simulink model "QubeServo3Disk_Workspace"  (R2023a)
settings: Solver=ode4  StartTime=0.0  StopTime=inf  FixedStep=1/1000  RelTol=1e-3  EnableMultiTasking=on
libraries: quarc_library x6, simulink x5
settings Model: SimulationMode=external  ExtModeTrigDuration=10000  Creator=mbohra  LastModifiedBy=mbohra
settings SolverCC: AlgebraicLoopSolver=TrustRegion  PositivePriorityOrder=on
settings DataIOCC: ReturnWorkspaceOutputs=off
settings OptimizationCC: ReuseModelBlockBuffer=off
settings DebuggingCC: UnconnectedInputMsg=warning  UnconnectedOutputMsg=warning  UnconnectedLineMsg=warning  ArithmeticOperatorsInVariantConditions=warning
settings ModelReferenceCC: EnableRefExpFcnMdlSchedulingChecks=on
settings SFSimCC: SimUseLocalCustomCode=off  CustomCodeUndefinedFunction=UseInterfaceOnly
settings RTWCC: Description=QUARC Win64 Target Using Toolchain  SystemTargetFile=quarc_win64.tlc  TemplateMakefile=quarc_default_tmf  RTWUseLocalCustomCode=off  Toolchain=QUARC win64 | nmake (64-bit Windows)  BuildConfiguration=Faster Runs  DLArmComputeVersion=19.05
settings CodeAppCC: StateflowObjectComments=on
settings STFCustomTargetCC: SystemTargetFile=quarc_win64.tlc
settings GRTTargetCC: ParMdlRefBuildCompliant=off  CompOptLevelCompliant=off  CombineOutputUpdateFcns=off  MatFileLogging=off  CPPClassGenCompliant=off  GRTInterface=on  ExtMode=on  ExtModeMexFile=quarc_comm
settings ConfigComp: CovMetricSettings=dswe

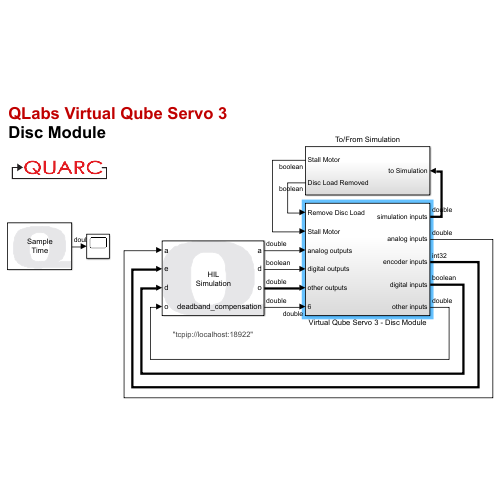
[thumbnail: Simulink's stored preview of the top-level diagram]
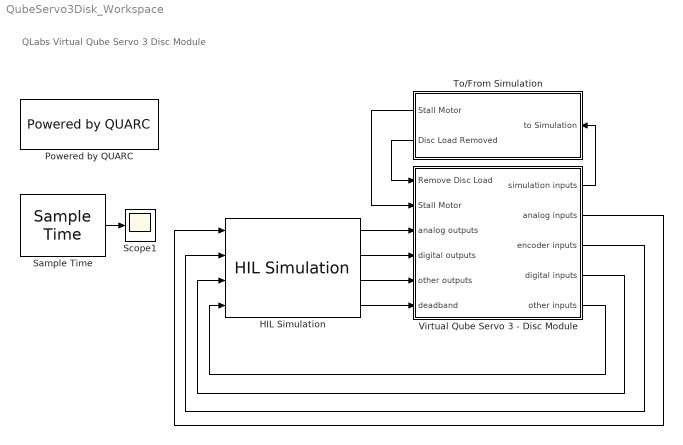
== system QubeServo3Disk_Workspace ==
  note: QLabs Virtual Qube Servo 3
      | Disc Module
  HIL Simulation : quarc_library/Data Acquisition/Generic/Configuration/HIL Simulation  uri_source=Specify via dialog (do not evaluate)  uri=tcpip://localhost:18922  board_type=qube_servo3_usb  board_id=0  options=deadband_compensation=%f[0,0.70]  sample_time=qc_get_step_size  active=on  num_clocks=1  num_interrupts=0  num_analog_inputs=1  num_analog_outputs=1  initial_analog=[]  num_digital_io=0  num_digital_inputs=3  num_digital_outputs=1  initial_digital=[]  num_encoder_inputs=2  num_pwm_outputs=0  initial_pwm=[]  other_inputs=[14000]  other_outputs=[11000:11002]  initial_other=[]  integer_get_property_codes=[]  double_get_property_codes=[]  string_get_property_codes=[]  integer_set_property_codes=[]  double_set_property_codes=[]  string_set_property_codes=[]  initial_integer_properties=0  initial_double_properties=0  max_string_property=80  use_variable_size_strings=off
      settings: AttributesFormatString="\"tcpip://localhost:18922\""  SourceProductName=QUARC Targets
  Powered by QUARC : quarc_library/Logos/Powered by QUARC
  Sample Time : quarc_library/Sources/Time/Sample Time  Priority=-99  sample_time=qc_get_step_size
  Scope1 : Scope
  To/From Simulation : Subsystem
  Virtual Qube Servo 3 - Disc Module : Subsystem
  wires:
  Sample Time/1 -> Scope1/1
  Virtual Qube Servo 3 - Disc Module/1(simulation inputs) -> To/From Simulation/1(to Simulation)
  HIL Simulation/1 -> Virtual Qube Servo 3 - Disc Module/3(analog outputs)
  HIL Simulation/2 -> Virtual Qube Servo 3 - Disc Module/4(digital outputs)
  Virtual Qube Servo 3 - Disc Module/2(analog inputs) -> HIL Simulation/1
  Virtual Qube Servo 3 - Disc Module/5(other inputs) -> HIL Simulation/4
  Virtual Qube Servo 3 - Disc Module/3(encoder inputs) -> HIL Simulation/2
  Virtual Qube Servo 3 - Disc Module/4(digital inputs) -> HIL Simulation/3
  To/From Simulation/2(Disc Load Removed) -> Virtual Qube Servo 3 - Disc Module/1(Remove Disc Load)
  To/From Simulation/1(Stall Motor) -> Virtual Qube Servo 3 - Disc Module/2(Stall Motor)
  HIL Simulation/3 -> Virtual Qube Servo 3 - Disc Module/5(other outputs)
  HIL Simulation/4 -> Virtual Qube Servo 3 - Disc Module/6(deadband)

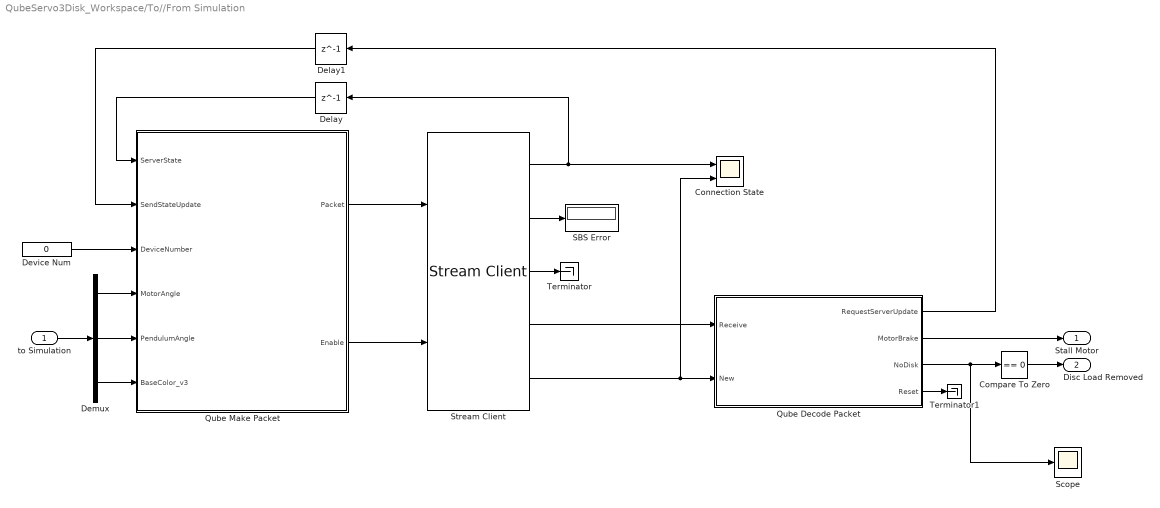
== system QubeServo3Disk_Workspace/To//From Simulation ==
  to Simulation : Inport
  Compare To Zero : simulink/Logic and Bit Operations/Compare To Zero  relop===  OutDataTypeStr=boolean
  "Connection State " : Scope  NumInputPorts=2
  Delay : Delay  DelayLength=1
  Delay1 : Delay  DelayLength=1
  Demux : Demux  Outputs=[1,1,3]
  Device Num : Constant  Value=0
  Qube Decode Packet : MATLAB Function  TreatAsAtomicUnit=on
  Qube Make Packet : MATLAB Function  TreatAsAtomicUnit=on
  SBS Error : Display
  Scope : Scope
  Stream Client : quarc_library/Communications/Basic/Stream Client  uri_source=Specify via dialog (do not evaluate)  uri=tcpip://localhost:18000?nagle='off'  send_buffer_size=65537  receive_buffer_size=65537  byte_order=little endian (Intel - LSB first)  optimization=Minimum latency  send_options=Send all data  receive_options=Receive all data  default_value=[0]  sample_time=qc_get_step_size  active=off  implementation=Use blocking I/O in a separate thread  send_fifo_size=3  receive_fifo_size=3  send_priority=0  receive_priority=0  send_dimensions=on  receive_dimensions=on  max_dimensions=65537  data_type=uint8  type_expr=BusObject
      settings: AttributesFormatString="\"tcpip://localhost:18000?nagle='off'\""
  Terminator : Terminator
  Terminator1 : Terminator
  Stall Motor : Outport  VectorParamsAs1DForOutWhenUnconnected=off
  Disc Load Removed : Outport  Port=2  VectorParamsAs1DForOutWhenUnconnected=off
  wires:
  Stream Client/4 -> Qube Decode Packet/1(Receive)
  Stream Client/5 -> "Connection State "/2, Qube Decode Packet/2(New)
  Stream Client/2 -> SBS Error/1
  Qube Decode Packet/1(RequestServerUpdate) -> Delay1/1
  Stream Client/3 -> Terminator/1
  Device Num/1 -> Qube Make Packet/3(DeviceNumber)
  Delay1/1 -> Qube Make Packet/2(SendStateUpdate)
  Delay/1 -> Qube Make Packet/1(ServerState)
  Stream Client/1 -> Delay/1, "Connection State "/1
  Qube Make Packet/1(Packet) -> Stream Client/1
  Qube Make Packet/2(Enable) -> Stream Client/2
  to Simulation/1 -> Demux/1
  Demux/1 -> Qube Make Packet/4(MotorAngle)
  Demux/2 -> Qube Make Packet/5(PendulumAngle)
  Demux/3 -> Qube Make Packet/6(BaseColor_v3)
  Qube Decode Packet/3(NoDisk) -> Scope/1, Compare To Zero/1
  Qube Decode Packet/4(Reset) -> Terminator1/1
  Qube Decode Packet/2(MotorBrake) -> Stall Motor/1
  Compare To Zero/1 -> Disc Load Removed/1

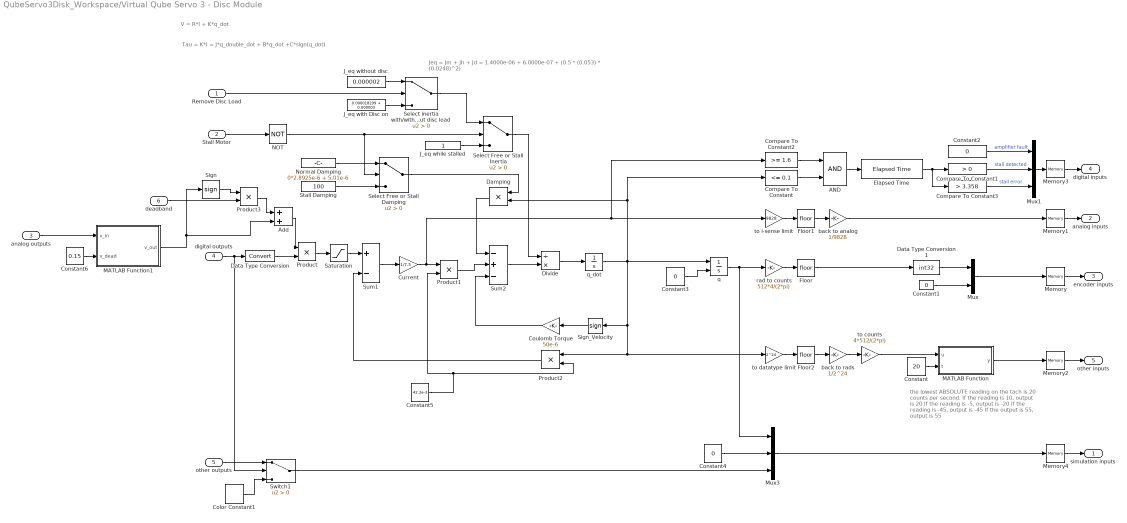
== system QubeServo3Disk_Workspace/Virtual Qube Servo 3 - Disc Module ==
  note: Jeq 		= Jm + Jh + Jd
      | 		= 1.4000e-06  +  6.0000e-07  +  (0.5 * (0.053) * (0.0248)^2)
  note: the lowest ABSOLUTE reading on the tach
      | is 20 counts per second.
      |
      | If the reading is 10, output is 20
      | If the reading is -5, output is -20
      | If the reading is -45, output is -45
      | If the output is 55, output is 55
  note: Tau = K*I = J*q_double_dot + B*q_dot +C*sign(q_dot)
  note: V = R*I + K*q_dot
  Remove Disc Load : Inport
  Stall Motor : Inport  Port=2
  analog outputs : Inport  Port=3
  digital outputs : Inport  Port=4
  other outputs : Inport  Port=5
  deadband : Inport  Port=6
  AND : Logic  AllPortsSameDT=off  OutDataTypeStr=boolean
  Add : Sum
  Color Constant1 : quarc_library/Sources/Signals/Color Constant  color=[1 0 0]
      settings: SourceProductName=QUARC Targets
  Compare To Constant : simulink/Logic and Bit Operations/Compare To Constant  relop=<=  const=0.1  OutDataTypeStr=boolean
  Compare To Constant1 : simulink/Logic and Bit Operations/Compare To Constant  relop=>  const=0  OutDataTypeStr=boolean
  Compare To Constant2 : simulink/Logic and Bit Operations/Compare To Constant  relop=>=  const=1.6  OutDataTypeStr=boolean
  Compare To Constant3 : simulink/Logic and Bit Operations/Compare To Constant  relop=>  const=3.358  OutDataTypeStr=boolean
  Constant : Constant  Value=20
  Constant1 : Constant  Value=0  OutDataTypeStr=int32
  Constant2 : Constant  Value=0  OutDataTypeStr=Inherit: Inherit via back propagation
  Constant3 : Constant  Value=0
  Constant4 : Constant  Value=0
  Constant5 : Constant  Value=42.2e-3
  Constant6 : Constant  Value=0.15
  Coulomb Torque : Gain  Gain=50e-6
  Current : Gain  Gain=1/7.5
  Damping : Product
  Data Type Conversion : DataTypeConversion  SaturateOnIntegerOverflow=off  RndMeth=Floor
  Data Type Conversion1 : DataTypeConversion  OutDataTypeStr=int32  SaturateOnIntegerOverflow=off  RndMeth=Floor
  Divide : Product  Inputs=/*
  Elapsed Time : quarc_library/Advanced/Timing/Elapsed Time  start_src=on  sample_time=-1
      settings: SourceProductName=QUARC Targets
  Floor : Rounding
  Floor1 : Rounding
  Floor2 : Rounding
  J_eq while stalled : Constant
  "J_eq with Disc on " : Constant  Value=0.000018299 + 0.000003
  J_eq without disc : Constant  Value=0.000002
  MATLAB Function : MATLAB Function  TreatAsAtomicUnit=on
  MATLAB Function1 : MATLAB Function  TreatAsAtomicUnit=on
  Memory : Memory  InitialCondition=[0 0]  InheritSampleTime=on
  Memory1 : Memory
  Memory2 : Memory
  Memory3 : Memory  InitialCondition=[0 0 0]
  Memory4 : Memory  InitialCondition=[0 0 1 0 0]
  Mux : Mux  Inputs=2
  Mux1 : Mux  Inputs=3
  Mux3 : Mux  Inputs=3
  NOT : Logic  Operator=NOT  IconShape=distinctive  AllPortsSameDT=off  OutDataTypeStr=boolean
  Normal Damping : Constant  Value=0*2.8925e-6 + 5.01e-6
  Product{,1..3} (4 alike) : Product
  Saturation : Saturate  UpperLimit=15  LowerLimit=-15
  Select Free or Stall Damping : Switch  Criteria=u2 > Threshold  SaturateOnIntegerOverflow=off  InputSameDT=off
  Select Free or Stall Inertia : Switch  Criteria=u2 > Threshold  SaturateOnIntegerOverflow=off  InputSameDT=off
  Select inertia with/without disc load : Switch  Criteria=u2 > Threshold  SaturateOnIntegerOverflow=off  InputSameDT=off
  Sign : Signum
  Sign_Velocity : Signum
  Stall Damping : Constant  Value=100
  Sum1 : Sum  Inputs=+-
  Sum2 : Sum  Inputs=-+-
  Switch1 : Switch  Criteria=u2 > Threshold  SaturateOnIntegerOverflow=off  InputSameDT=off
  back to rads : Gain  Gain=1/2^24
  back to analog : Gain  Gain=1/9828
  q : Integrator  ExternalReset=either
  q_dot : Integrator
  rad to counts : Gain  Gain=512*4/(2*pi)
  to counts : Gain  Gain=4*512/(2*pi)
  to datatype limit : Gain  Gain=2^24
  to i-sense limit : Gain  Gain=9828
  simulation inputs : Outport  VectorParamsAs1DForOutWhenUnconnected=off
  analog inputs : Outport  Port=2  VectorParamsAs1DForOutWhenUnconnected=off
  encoder inputs : Outport  Port=3  VectorParamsAs1DForOutWhenUnconnected=off
  digital inputs : Outport  Port=4  VectorParamsAs1DForOutWhenUnconnected=off
  other inputs : Outport  Port=5  VectorParamsAs1DForOutWhenUnconnected=off
  wires:
  digital outputs/1 -> Switch1/2, Data Type Conversion/1
  rad to counts/1 -> Floor/1
  q/1 -> Mux3/1, rad to counts/1
  Mux/1 -> Memory/1
  Constant1/1 -> Mux/2
  Data Type Conversion/1 -> Product/2
  Data Type Conversion1/1 -> Mux/1
  Memory/1 -> encoder inputs/1
  Memory1/1 -> analog inputs/1
  Memory2/1 -> other inputs/1
  Mux1/1 -> Memory3/1
  Compare To Constant/1 -> AND/2
  Compare To Constant2/1 -> AND/1
  AND/1 -> Elapsed Time/1
  Elapsed Time/1 -> Compare To Constant1/1, Compare To Constant3/1
  Compare To Constant1/1 -> Mux1/2  "stall detected"
  Compare To Constant3/1 -> Mux1/3  "stall error"
  Constant2/1 -> Mux1/1  "amplifier fault"
  Memory3/1 -> digital inputs/1
  Floor/1 -> Data Type Conversion1/1
  to counts/1 -> MATLAB Function/1(u)
  to datatype limit/1 -> Floor2/1
  Floor2/1 -> back to rads/1
  back to rads/1 -> to counts/1
  MATLAB Function/1(y) -> Memory2/1
  to i-sense limit/1 -> Floor1/1
  Floor1/1 -> back to analog/1
  back to analog/1 -> Memory1/1
  Constant/1 -> MATLAB Function/2(t)
  Constant3/1 -> q/2
  Saturation/1 -> Sum1/1
  q_dot/1 -> Compare To Constant/1, Damping/2, Product2/1, to datatype limit/1, Sign_Velocity/1, q/1
  Sum2/1 -> Divide/2
  Coulomb Torque/1 -> Sum2/3
  Divide/1 -> q_dot/1
  Sign_Velocity/1 -> Coulomb Torque/1
  Product2/1 -> Sum1/2
  Current/1 -> Product1/1, to i-sense limit/1, Compare To Constant2/1
  Product/1 -> Saturation/1
  Sum1/1 -> Current/1
  Product1/1 -> Sum2/2
  Select inertia with/without disc load/1 -> Select Free or Stall Inertia/1
  Stall Motor/1 -> NOT/1
  J_eq while stalled/1 -> Select Free or Stall Inertia/3
  J_eq without disc/1 -> Select inertia with/without disc load/1
  "J_eq with Disc on "/1 -> Select inertia with/without disc load/3
  Select Free or Stall Inertia/1 -> Divide/1
  other outputs/1 -> Switch1/1
  Constant4/1 -> Mux3/2
  Mux3/1 -> Memory4/1
  Color Constant1/1 -> Switch1/3
  Memory4/1 -> simulation inputs/1
  Switch1/1 -> Mux3/3
  Damping/1 -> Sum2/1
  Stall Damping/1 -> Select Free or Stall Damping/3
  Normal Damping/1 -> Select Free or Stall Damping/1
  Select Free or Stall Damping/1 -> Damping/1
  NOT/1 -> Select Free or Stall Damping/2, Select Free or Stall Inertia/2
  Constant5/1 -> Product2/2, Product1/2
  MATLAB Function1/1(v_out) -> Add/2, Sign/1
  Sign/1 -> Product3/1
  deadband/1 -> Product3/2
  Product3/1 -> Add/1
  Add/1 -> Product/1
  Remove Disc Load/1 -> Select inertia with/without disc load/2
  Constant6/1 -> MATLAB Function1/2(v_dead)
  analog outputs/1 -> MATLAB Function1/1(v_in)

== matlab function QubeServo3Disk_Workspace/To//From Simulation/Qube Make Packet ==
  settings: updateMethod=DISCRETE  sampleTime=qc_get_step_size
  data: Packet output size=65537; ServerState input; SendStateUpdate input; Enable output; DeviceNumber input; MotorAngle input; PendulumAngle input; BaseColor_v3 input
function [Packet,Enable] = QubeMakePacket(ServerState, SendStateUpdate, DeviceNumber, MotorAngle, PendulumAngle, BaseColor_v3) 

% Be sure to set the maximum signal size of the variable size Packet port 
% in Simulink->Edit Data of the editor window.  Size should be 65537 or
% larger to ensure that the stream server generates a 4 byte packet size.

%% Setup
persistent LastServerState;

if isempty(LastServerState)
    LastServerState = uint8(0);
end

Enable = 0;
Packet = uint8([]);

%% On connection
if ((ServerState == 2) && (LastServerState ~= 2))
    Packet = Qube3MakeCommandStateContainer(DeviceNumber, MotorAngle, PendulumAngle, BaseColor_v3); 
    Packet = [Packet; Qube3MakeModeRequestContainer(DeviceNumber)];
end

%% Send new State Container
% Previous state processed, send a new one
if (SendStateUpdate)
    Packet = Qube3MakeCommandStateContainer(DeviceNumber, MotorAngle, PendulumAngle, BaseColor_v3); 
end

%% Transmit
% If we have data to send, enable the transmit
PacketLength = length(Packet);

if (PacketLength > 0)
    % Add magic byte.  This is just for error handling and isn't typically
    % required in simulink, but useful in lower-level languages like Python
    Packet = [uint8(123); Packet];
    
    Enable = 1; 
end


LastServerState = ServerState;

== matlab function QubeServo3Disk_Workspace/Virtual Qube Servo 3 - Disc Module/MATLAB Function ==
  data: u input; y output; t input
function y = tach_model(u, t)

y = u;

if (u >= 0)&&(u < t)
    y = t;
elseif (u < 0)&&(u > -t)
    y = -t;
end

== matlab function QubeServo3Disk_Workspace/To//From Simulation/Qube Decode Packet ==
  data: Receive input size=65537; RequestServerUpdate output; New input; MotorBrake output; NoDisk output; Reset output
function [RequestServerUpdate, MotorBrake, NoDisk, Reset] = QubeDecodePacket(Receive, New)

%% Setup

persistent iMotorBrake;
persistent iQubeMode;

if isempty(iQubeMode)
    iMotorBrake = uint8(0);
    iQubeMode = uint8(0);
end

% Need to assign outputs here even though they are reassigned at the end
% since matlab can't determine the signal widths
MotorBrake = false;
NoDisk = uint8(0);
Reset = 0;
RequestServerUpdate = 0;

PacketSize = length(Receive);

% Packet > 0, new data, and magic number in first index
if ((PacketSize > 0) && (New == 1) && (Receive(1) == uint8(123)))
    
    %skip magic number
    Index = int32(2);
    
    while(Index <= PacketSize)        
        
        %% Get container details
        ContainerSize = typecast(uint8(flip(Receive(Index:Index+3))), 'int32');
        DeviceID = typecast(uint8(flip(Receive(Index+4:Index+7))), 'int32');
        DeviceNum = typecast(uint8(flip(Receive(Index+8:Index+11))), 'int32');
        DeviceFunction = uint8(Receive(Index+12));
        PayloadStart = Index+13;
        PayloadEnd = Index+ContainerSize-1;
        
        %% Pass container to appropriate decoding function
        if (DeviceID == 61) %is this a Qube2 container?
            
            if (DeviceFunction == 11) %UE4 State Response
                iMotorBrake = uint8(Receive(PayloadStart));
                RequestServerUpdate = 1;
            elseif (DeviceFunction == 13) %Mode change
                iQubeMode = uint8(Receive(PayloadStart)); 
            end
        
        elseif (DeviceID == 1001) %Simulink notification
            if (DeviceFunction == 200) %Reset button
                Reset = 1;
            end
        end
        
        
        
        %% Process next container if any data is left.
        Index = Index+ContainerSize;
    end


end

MotorBrake = (iMotorBrake > 0);
NoDisk = iQubeMode;

== matlab function QubeServo3Disk_Workspace/Virtual Qube Servo 3 - Disc Module/MATLAB Function1 ==
  data: v_in input; v_out output; v_dead input
function v_out = fcn(v_in, v_dead)
v_out = v_in;
if abs(v_in) < v_dead
    v_out = 0;
end
end
